simulink model "BlueROV2_Exp_Simu"  (R2023b)
settings: Solver=FixedStepAuto  StartTime=0.0  StopTime=120  FixedStep=dt  RelTol=1e-3
values from neighbouring files (symbols this model uses):
  Af = diag(ti)    [RM_param_AGF.m]
  B = [zeros(6,6) ... (first row only)    [EKF_param.m]
  Ballast_Force = Ballast_Compute(Ballast_Config)    [Integrate.m]    (also in init.m = Ballast_Term(Ballast_Config); init_NIF.m = [0; 0; 0; 0; 0; 0]; init_NIF2.m = [0; 0; Ballast_Term; 0]; init_ODE.m)
  dt = 0.1    [Integrate.m]    (also in init.m; init_NIF.m; init_NIF2.m; init_ODE.m)
  Gamma = diag(omega_is)    [RM_param_AGF.m]
  Gamma_o = dt*E    [EKF_param.m]
  H = [eye(6), zeros(6,6) zeros(6,6)]    [EKF_param.m]
  inv_M = inv(Param.MT)    [EKF_param.m]
  inv_Tb = inv(Tb)    [EKF_param.m]
  Kd = [155; 355; 8985; 1205; 1205; 1]    [Integrate.m]    (also in init.m = [1; 1; 1; 1; 1; 1]; init_NIF.m; init_NIF2.m; init_ODE.m)
  Ki = [45; 45; 10; 96; 96; 1]    [Integrate.m]    (also in init.m = [1; 1; 1; 1; 1; 1]; init_NIF.m; init_NIF2.m; init_ODE.m)
  Kp = [255; 545; 7095; 2420; 2375; 1]    [Integrate.m]    (also in init.m = [1; 1; 1; 1; 1; 1]; init_NIF.m; init_NIF2.m; init_ODE.m)
  lower_limit = -upper_limit    (= -30)    [Integrate.m]    (also in init.m; init_NIF.m; init_NIF2.m; init_ODE.m)
  Omega = diag(2*omega_is.*zeta_is)    [RM_param_AGF.m]
  Param = BlueROV2_param()    [Integrate.m]    (also in init.m; init_NIF.m; init_NIF2.m; init_ODE.m)
  Q = diag([0.1,0.1,pi/180,1e6,1e6,1e9])*10e3    [EKF_param.m]
  R = diag([0.00001,0.00001,0.00001,      0.01*pi/180,0.01*pi/180,0.01*pi/180])*10e-4    [EKF_param.m]
  T_alloc = Thrust_Allocation()    [Integrate.m]    (also in init_NIF.m; init_NIF2.m; init_ODE.m; init_ballast_checking.m)
  T_alloc_ps = pinv(T_alloc' * T_alloc + lambda * eye(size(T_alloc, 2))) * T_alloc'    [Integrate.m]    (also in init_NIF.m; init_NIF2.m; init_ODE.m; init_ballast_checking.m)
  Tether_Force = zeros(6,1)    [Integrate.m]    (also in init.m; init_NIF.m; init_NIF2.m; init_ODE.m)
  thrust_rate = 5    [Integrate.m]    (also in init.m; init_NIF.m; init_NIF2.m; init_ODE.m)
  upper_limit = 30    [Integrate.m]    (also in init.m; init_NIF.m; init_NIF2.m; init_ODE.m)
undefined symbols (not defined in the file or in its folder): model_val, Phi_ref, Psi_ref, Theta_ref, time_stamps_phi, time_stamps_psi, time_stamps_theta, time_stamps_x, time_stamps_y, time_stamps_z, time_val, X_ref, Y_ref, Z_ref
libraries: slpidlib x6
(part 1 of 2)
settings Model: Creator=goks  LastModifiedBy=HP

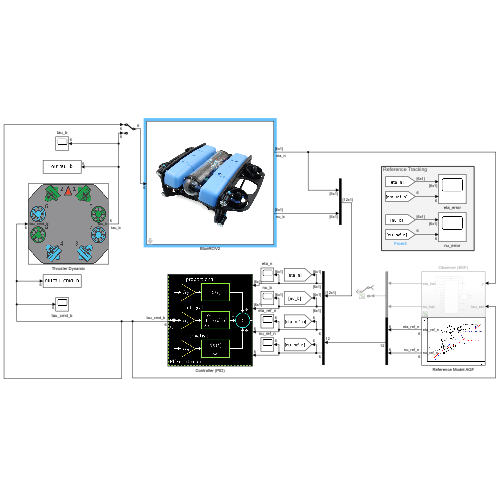
[thumbnail: Simulink's stored preview of the top-level diagram]
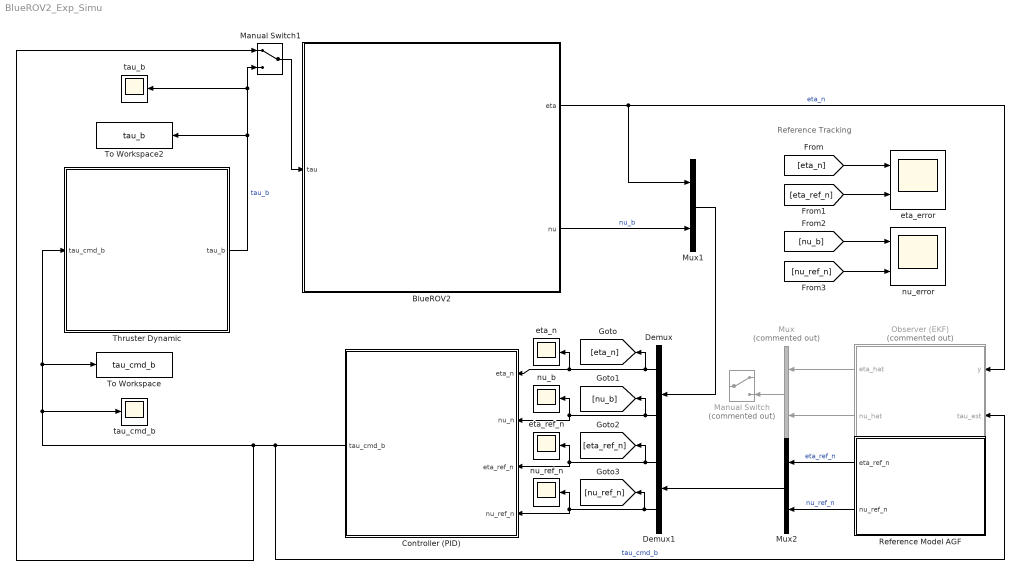
== system BlueROV2_Exp_Simu ==
  note: Reference Tracking
  BlueROV2 : Subsystem
      mask DialogControl DescTextVar Prompt: %<BlueROV2>
      mask Display: image('heavy-bluerov.jpg');
  Controller (PID) : Subsystem
      mask Display: image('pid.jpeg');
  Demux : Demux  Outputs=2
  Demux1 : Demux  Outputs=2
  Manual Switch : ManualSwitch  Commented=on
  Manual Switch1 : ManualSwitch
  Mux : Mux  Commented=on  Inputs=2
  Mux1 : Mux  Inputs=2
  Mux2 : Mux  Inputs=2
  Observer (EKF) : Subsystem  Commented=on
  Reference Model AGF : Subsystem
      mask Display: image('ref_traj_img.png');
  Thruster Dynamic : Subsystem
      mask Display: image('blueROV2_heavy_config.png');
  To Workspace : ToWorkspace  VariableName=tau_cmd_b  SampleTime=-1
  To Workspace2 : ToWorkspace  VariableName=tau_b  SampleTime=-1
  eta_error : Scope  NumInputPorts=2
  eta_n : Scope
  eta_ref_n : Scope
  nu_b : Scope
  nu_error : Scope  NumInputPorts=2
  nu_ref_n : Scope
  tau_b : Scope
  tau_cmd_b : Scope
  wires:
  BlueROV2/1(eta) -> Observer (EKF)/1(y), Mux1/1  "eta_n"
  Thruster Dynamic/1(tau_b) -> tau_b/1, Manual Switch1/2, To Workspace2/1  "tau_b"
  Controller (PID)/1(tau_cmd_b) -> Thruster Dynamic/1(tau_cmd_b), To Workspace/1, tau_cmd_b/1, Manual Switch1/1, Observer (EKF)/2(tau_est)  "tau_cmd_b"
  Observer (EKF)/1(eta_hat) -> Mux/1
  Observer (EKF)/2(nu_hat) -> Mux/2
  Mux/1 -> Manual Switch/2
  BlueROV2/2(nu) -> Mux1/2  "nu_b"
  Mux1/1 -> Demux/1
  Demux/1 -> Controller (PID)/1(eta_n), eta_n/1, [eta_n]
  Demux/2 -> Controller (PID)/2(nu_n), nu_b/1, [nu_b]
  Mux2/1 -> Demux1/1
  Demux1/1 -> Controller (PID)/3(eta_ref_n), eta_ref_n/1, [eta_ref_n]
  Demux1/2 -> Controller (PID)/4(nu_ref_n), nu_ref_n/1, [nu_ref_n]
  Manual Switch1/1 -> BlueROV2/1(tau)
  Reference Model AGF/1(eta_ref_n) -> Mux2/1  "eta_ref_n"
  Reference Model AGF/2(nu_ref_n) -> Mux2/2  "nu_ref_n"
  [eta_n] -> eta_error/1
  [eta_ref_n] -> eta_error/2
  [nu_b] -> nu_error/1
  [nu_ref_n] -> nu_error/2

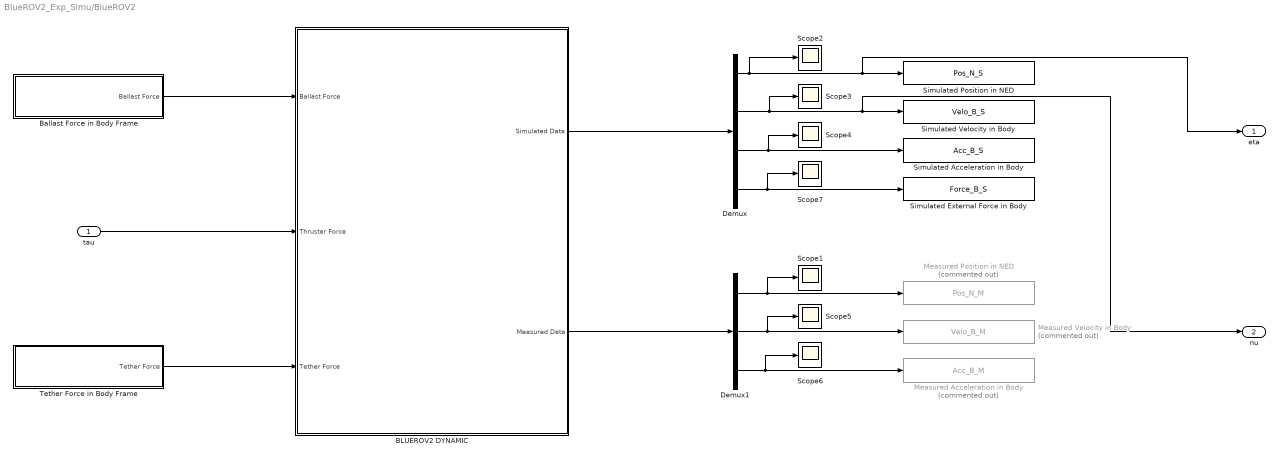
== system BlueROV2_Exp_Simu/BlueROV2 ==
  tau : Inport
  BLUEROV2 DYNAMIC : Subsystem
  Ballast Force in Body Frame : Subsystem
  Demux : Demux
  Demux1 : Demux  Outputs=3
  Measured Acceleration in Body : ToWorkspace  Commented=on  VariableName=Acc_B_M  SampleTime=-1
  Measured Position in NED : ToWorkspace  Commented=on  VariableName=Pos_N_M  SampleTime=-1
  Measured Velocity in Body : ToWorkspace  Commented=on  VariableName=Velo_B_M  SampleTime=-1
  Scope{1..7} (7 alike) : Scope
  Simulated Acceleration in Body : ToWorkspace  VariableName=Acc_B_S  SampleTime=-1
  Simulated External Force in Body : ToWorkspace  VariableName=Force_B_S  SampleTime=-1
  Simulated Position in NED : ToWorkspace  VariableName=Pos_N_S  SampleTime=-1
  Simulated Velocity in Body : ToWorkspace  VariableName=Velo_B_S  SampleTime=-1
  Tether Force in Body Frame : Subsystem
  eta : Outport
  nu : Outport  Port=2
  wires:
  Tether Force in Body Frame/1(Tether Force) -> BLUEROV2 DYNAMIC/3(Tether Force)
  Demux/2 -> nu/1, Simulated Velocity in Body/1, Scope3/1
  BLUEROV2 DYNAMIC/1(Simulated Data) -> Demux/1
  Demux1/1 -> Measured Position in NED/1, Scope1/1
  BLUEROV2 DYNAMIC/2(Measured Data) -> Demux1/1
  Ballast Force in Body Frame/1(Ballast Force) -> BLUEROV2 DYNAMIC/1(Ballast Force)
  Demux/1 -> eta/1, Simulated Position in NED/1, Scope2/1
  Demux/3 -> Simulated Acceleration in Body/1, Scope4/1
  tau/1 -> BLUEROV2 DYNAMIC/2(Thruster Force)
  Demux1/2 -> Measured Velocity in Body/1, Scope5/1
  Demux1/3 -> Scope6/1, Measured Acceleration in Body/1
  Demux/4 -> Scope7/1, Simulated External Force in Body/1

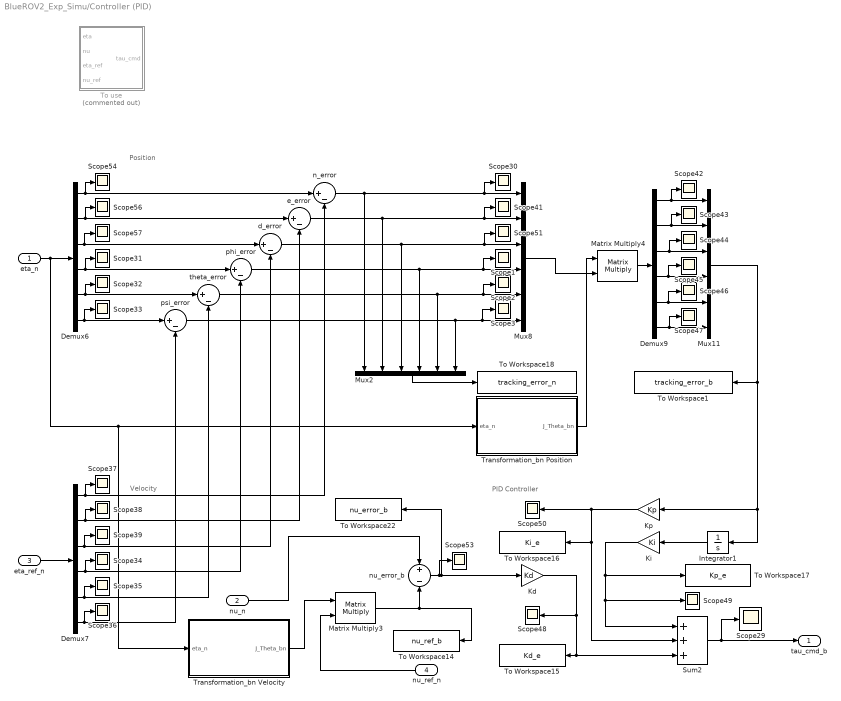
== system BlueROV2_Exp_Simu/Controller (PID) ==
  note: Velocity
  note: Position
  note: PID Controller
  eta_n : Inport
  nu_n : Inport  Port=2
  eta_ref_n : Inport  Port=3
  nu_ref_n : Inport  Port=4
  Demux6 : Demux  Outputs=6
  Demux7 : Demux  Outputs=6
  Demux9 : Demux  Outputs=6
  Integrator1 : Integrator
  Kd : Gain  Gain=Kd
  Ki : Gain  Gain=Ki
  Kp : Gain  Gain=Kp
  Matrix Multiply3 : Product  Multiplication=Matrix(*)
  Matrix Multiply4 : Product  Multiplication=Matrix(*)
  Mux11 : Mux  Inputs=6
  Mux2 : Mux  Inputs=6
  Mux8 : Mux  Inputs=6
  Scope{1..3,29..39,41..51,53..54,56..57} (29 alike) : Scope
  Sum2 : Sum  Inputs=+++
  To Workspace1 : ToWorkspace  VariableName=tracking_error_b  SampleTime=-1
  To Workspace14 : ToWorkspace  VariableName=nu_ref_b  SampleTime=-1
  To Workspace15 : ToWorkspace  VariableName=Kd_e  SampleTime=-1
  To Workspace16 : ToWorkspace  VariableName=Ki_e  SampleTime=-1
  To Workspace17 : ToWorkspace  VariableName=Kp_e  SampleTime=-1
  To Workspace18 : ToWorkspace  VariableName=tracking_error_n  SampleTime=-1
  To Workspace22 : ToWorkspace  VariableName=nu_error_b  SampleTime=-1
  To use : Subsystem  Commented=on
  Transformation_bn Position : MATLAB Function  TreatAsAtomicUnit=on
  Transformation_bn Velocity : MATLAB Function  TreatAsAtomicUnit=on
  d_error : Sum  Inputs=|+-
  e_error : Sum  Inputs=|+-
  n_error : Sum  Inputs=|+-
  nu_error_b : Sum  Inputs=+|-
  phi_error : Sum  Inputs=|+-
  psi_error : Sum  Inputs=|+-
  theta_error : Sum  Inputs=|+-
  tau_cmd_b : Outport
  wires:
  nu_ref_n/1 -> Matrix Multiply3/2
  Demux6/5 -> theta_error/1, Scope32/1
  Sum2/1 -> Scope29/1, tau_cmd_b/1
  Matrix Multiply4/1 -> Demux9/1
  Transformation_bn Velocity/1(J_Theta_bn) -> Matrix Multiply3/1
  n_error/1 -> Scope30/1, Mux8/1, Mux2/1
  Matrix Multiply3/1 -> nu_error_b/2, To Workspace14/1
  Mux2/1 -> To Workspace18/1
  Demux9/2 -> Scope43/1, Mux11/2
  Demux6/6 -> psi_error/1, Scope33/1
  Demux7/1 -> Scope37/1, n_error/2
  Integrator1/1 -> Ki/1
  eta_ref_n/1 -> Demux7/1
  Demux9/6 -> Scope47/1, Mux11/6
  Mux11/1 -> Integrator1/1, Kp/1, To Workspace1/1
  e_error/1 -> Scope41/1, Mux8/2, Mux2/2
  Demux9/3 -> Scope44/1, Mux11/3
  Mux8/1 -> Matrix Multiply4/2
  Demux7/4 -> Scope34/1, phi_error/2
  Demux6/4 -> phi_error/1, Scope31/1
  Demux6/2 -> Scope56/1, e_error/1
  d_error/1 -> Scope51/1, Mux8/3, Mux2/3
  Ki/1 -> Scope49/1, Sum2/1, To Workspace17/1
  Demux9/5 -> Scope46/1, Mux11/5
  Demux6/1 -> Scope54/1, n_error/1
  Kp/1 -> Scope50/1, To Workspace16/1, Sum2/2
  Demux9/4 -> Scope45/1, Mux11/4
  Kd/1 -> Sum2/3, To Workspace15/1, Scope48/1
  nu_error_b/1 -> Kd/1, To Workspace22/1, Scope53/1
  Transformation_bn Position/1(J_Theta_bn) -> Matrix Multiply4/1
  Demux7/6 -> Scope36/1, psi_error/2
  Demux9/1 -> Scope42/1, Mux11/1
  nu_n/1 -> nu_error_b/1
  Demux6/3 -> Scope57/1, d_error/1
  Demux7/2 -> Scope38/1, e_error/2
  phi_error/1 -> Scope1/1, Mux8/4, Mux2/4
  theta_error/1 -> Mux8/5, Scope2/1, Mux2/5
  psi_error/1 -> Scope3/1, Mux8/6, Mux2/6
  Demux7/3 -> d_error/2, Scope39/1
  Demux7/5 -> Scope35/1, theta_error/2
  eta_n/1 -> Transformation_bn Position/1(eta_n), Transformation_bn Velocity/1(eta_n), Demux6/1

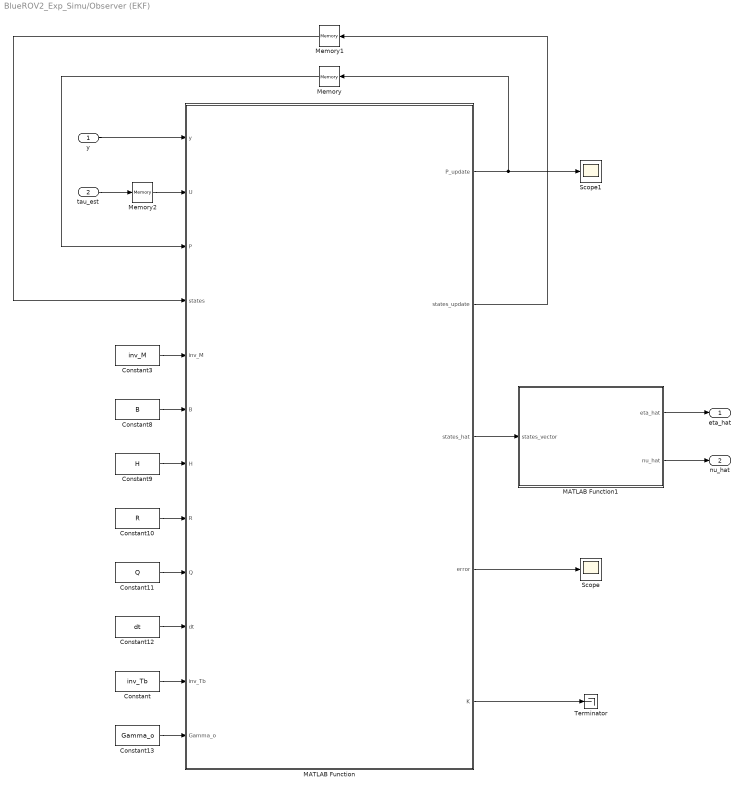
== system BlueROV2_Exp_Simu/Observer (EKF) ==
  y : Inport
  tau_est : Inport  Port=2
  Constant : Constant  Value=inv_Tb
  Constant10 : Constant  Value=R
  Constant11 : Constant  Value=Q
  Constant12 : Constant  Value=dt
  Constant13 : Constant  Value=Gamma_o
  Constant3 : Constant  Value=inv_M
  Constant8 : Constant  Value=B
  Constant9 : Constant  Value=H
  MATLAB Function : MATLAB Function  TreatAsAtomicUnit=on
  MATLAB Function1 : MATLAB Function  TreatAsAtomicUnit=on
  Memory : Memory  InitialCondition=eye(18)
  Memory1 : Memory  InitialCondition=zeros(18,1)
  Memory2 : Memory  InitialCondition=zeros(6,1)
  Scope : Scope
  Scope1 : Scope
  Terminator : Terminator
  eta_hat : Outport
  nu_hat : Outport  Port=2
  wires:
  y/1 -> MATLAB Function/1(y)
  Constant3/1 -> MATLAB Function/5(inv_M)
  Constant8/1 -> MATLAB Function/6(B)
  Constant9/1 -> MATLAB Function/7(H)
  Constant10/1 -> MATLAB Function/8(R)
  Constant11/1 -> MATLAB Function/9(Q)
  Constant12/1 -> MATLAB Function/10(dt)
  Constant/1 -> MATLAB Function/11(inv_Tb)
  Constant13/1 -> MATLAB Function/12(Gamma_o)
  MATLAB Function/1(P_update) -> Scope1/1, Memory/1
  Memory/1 -> MATLAB Function/3(P)
  MATLAB Function/2(states_update) -> Memory1/1
  Memory1/1 -> MATLAB Function/4(states)
  MATLAB Function/5(K) -> Terminator/1
  MATLAB Function/4(error) -> Scope/1
  MATLAB Function/3(states_hat) -> MATLAB Function1/1(states_vector)
  MATLAB Function1/1(eta_hat) -> eta_hat/1
  MATLAB Function1/2(nu_hat) -> nu_hat/1
  tau_est/1 -> Memory2/1
  Memory2/1 -> MATLAB Function/2(U)

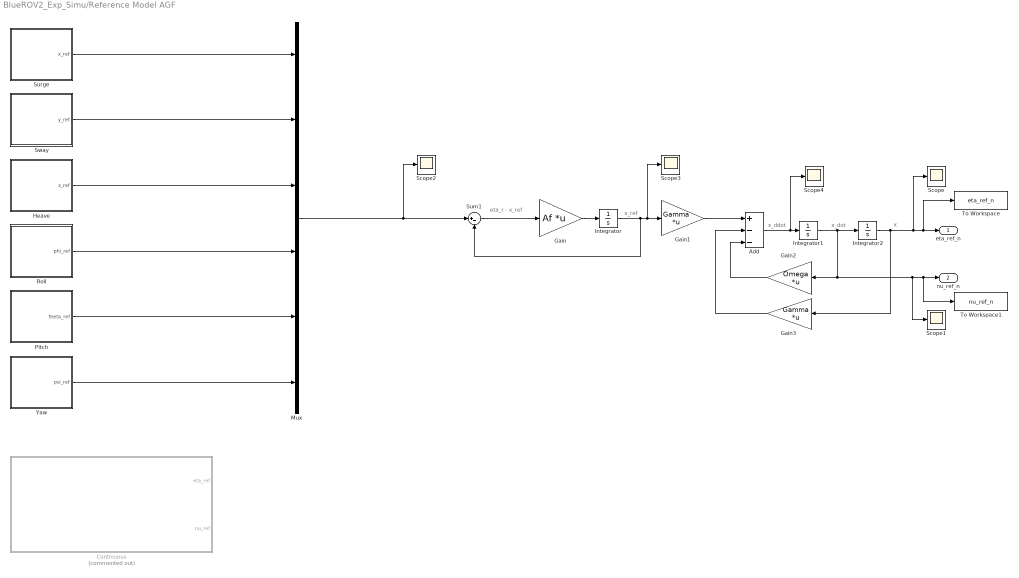
== system BlueROV2_Exp_Simu/Reference Model AGF ==
  note: x_dot
  note: eta_r - x_ref
  note: x
  note: x_ref
  note: x_ddot
  Add : Sum  Inputs=+--
  Continuous : Subsystem  Commented=on
  Gain : Gain  Gain=Af  Multiplication=Matrix(K*u)
  Gain1 : Gain  Gain=Gamma  Multiplication=Matrix(K*u)
  Gain2 : Gain  Gain=Omega  Multiplication=Matrix(K*u)
  Gain3 : Gain  Gain=Gamma  Multiplication=Matrix(K*u)
  Heave : Subsystem
  Integrator : Integrator
  Integrator1 : Integrator
  Integrator2 : Integrator
  Mux : Mux  Inputs=6
  Pitch : Subsystem
  Roll : Subsystem
  Scope{,1..4} (5 alike) : Scope
  Sum1 : Sum  Inputs=|+-
  Surge : Subsystem
  Sway : Subsystem
  To Workspace : ToWorkspace  VariableName=eta_ref_n  SampleTime=-1
  To Workspace1 : ToWorkspace  VariableName=nu_ref_n  SampleTime=-1
  Yaw : Subsystem
  eta_ref_n : Outport
  nu_ref_n : Outport  Port=2
  wires:
  Surge/1(x_ref) -> Mux/1
  Heave/1(z_ref) -> Mux/3
  Pitch/1(theta_ref) -> Mux/5
  Yaw/1(psi_ref) -> Mux/6
  Sway/1(y_ref) -> Mux/2
  Roll/1(phi_ref) -> Mux/4
  Gain1/1 -> Add/1
  Gain/1 -> Integrator/1
  Sum1/1 -> Gain/1
  Integrator1/1 -> Integrator2/1, To Workspace1/1, nu_ref_n/1, Scope1/1, Gain2/1
  Gain3/1 -> Add/2
  Integrator2/1 -> To Workspace/1, eta_ref_n/1, Scope/1, Gain3/1
  Gain2/1 -> Add/3
  Mux/1 -> Scope2/1, Sum1/1
  Integrator/1 -> Scope3/1, Gain1/1, Sum1/2
  Add/1 -> Scope4/1, Integrator1/1

== system BlueROV2_Exp_Simu/Thruster Dynamic ==
  tau_cmd_b : Inport
  Gain : Gain  Gain=T_alloc_ps  Multiplication=Matrix(K*u) (u vector)
  Gain1 : Gain  Gain=T_alloc  Multiplication=Matrix(K*u) (u vector)
  Manual Switch : ManualSwitch
  Saturation and Dynamics : Subsystem
      mask Display: image('t200-img.jpg');
  tau_b : Outport
  wires:
  Manual Switch/1 -> Gain1/1
  tau_cmd_b/1 -> Gain/1
  Saturation and Dynamics/1(Actual Thrust) -> Manual Switch/1
  Gain/1 -> Saturation and Dynamics/1(Commanded Thrust), Manual Switch/2
  Gain1/1 -> tau_b/1

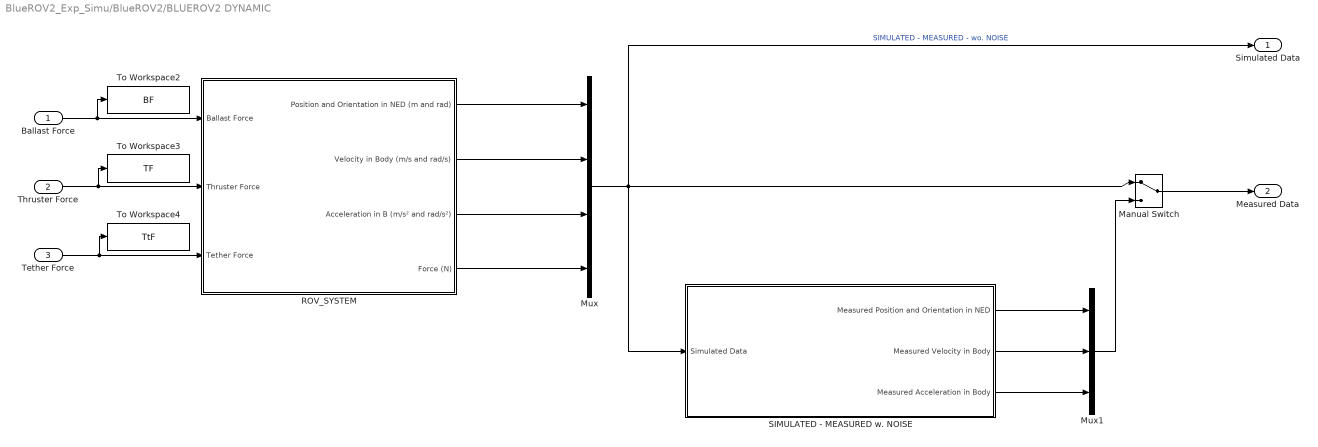
== system BlueROV2_Exp_Simu/BlueROV2/BLUEROV2 DYNAMIC ==
  Ballast Force : Inport
  Thruster Force : Inport  Port=2
  Tether Force : Inport  Port=3
  Manual Switch : ManualSwitch
  Mux : Mux
  Mux1 : Mux  Inputs=3
  ROV_SYSTEM : Subsystem
  SIMULATED - MEASURED w. NOISE : Subsystem
  To Workspace2 : ToWorkspace  VariableName=BF  SampleTime=-1
  To Workspace3 : ToWorkspace  VariableName=TF  SampleTime=-1
  To Workspace4 : ToWorkspace  VariableName=TtF  SampleTime=-1
  Simulated Data : Outport
  Measured Data : Outport  Port=2
  wires:
  ROV_SYSTEM/1(Position and Orientation in NED (m and rad)) -> Mux/1
  ROV_SYSTEM/2(Velocity in Body (m/s and rad/s)) -> Mux/2
  ROV_SYSTEM/3(Acceleration in B (m/s² and rad/s²)) -> Mux/3
  ROV_SYSTEM/4(Force (N)) -> Mux/4
  SIMULATED - MEASURED w. NOISE/2(Measured Velocity in Body) -> Mux1/2
  SIMULATED - MEASURED w. NOISE/1(Measured Position and Orientation in NED) -> Mux1/1
  SIMULATED - MEASURED w. NOISE/3(Measured Acceleration in Body) -> Mux1/3
  Mux/1 -> SIMULATED - MEASURED w. NOISE/1(Simulated Data), Manual Switch/1, Simulated Data/1  "SIMULATED - MEASURED - wo. NOISE"
  Manual Switch/1 -> Measured Data/1
  Mux1/1 -> Manual Switch/2
  Ballast Force/1 -> ROV_SYSTEM/1(Ballast Force), To Workspace2/1
  Thruster Force/1 -> ROV_SYSTEM/2(Thruster Force), To Workspace3/1
  Tether Force/1 -> To Workspace4/1, ROV_SYSTEM/3(Tether Force)

== system BlueROV2_Exp_Simu/BlueROV2/Ballast Force in Body Frame ==
  Ballast : Step  Time=0  Before=zeros(6,1)  After=Ballast_Force  SampleTime=0
  Scope : Scope
  Ballast Force : Outport
  wires:
  Ballast/1 -> Scope/1, Ballast Force/1

== system BlueROV2_Exp_Simu/BlueROV2/Tether Force in Body Frame ==
  Scope : Scope
  Tether : Step  Before=zeros(6,1)  After=Tether_Force  SampleTime=0
  Tether Force : Outport
  wires:
  Tether/1 -> Scope/1, Tether Force/1

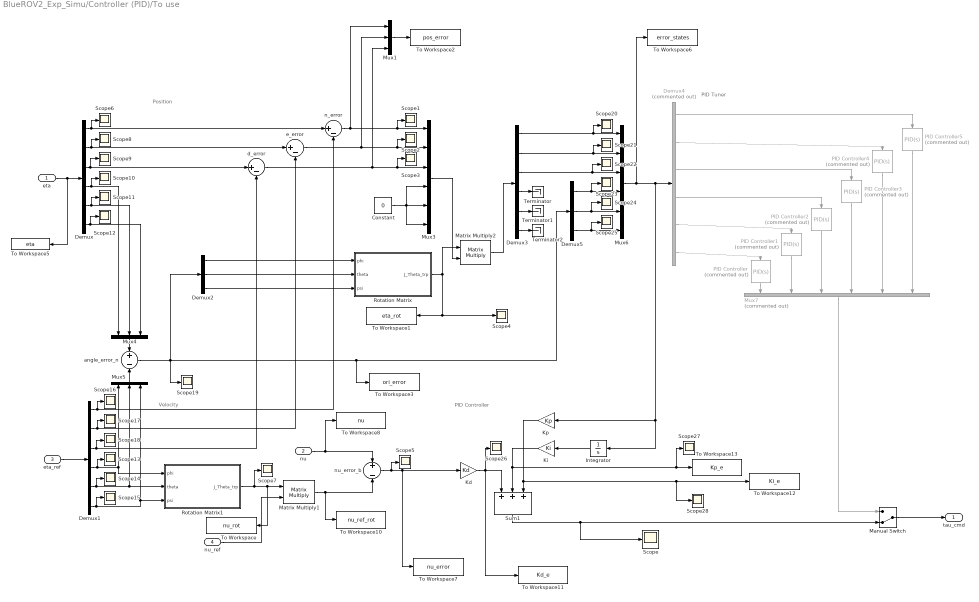
== system BlueROV2_Exp_Simu/Controller (PID)/To use ==
  note: PID Controller
  note: Velocity
  note: Position
  note: PID Tuner
  eta : Inport
  nu : Inport  Port=2
  eta_ref : Inport  Port=3
  nu_ref : Inport  Port=4
  Constant : Constant  Value=0
  Demux : Demux  Outputs=6
  Demux1 : Demux  Outputs=6
  Demux2 : Demux  Outputs=3
  Demux3 : Demux  Outputs=6
  Demux4 : Demux  Commented=on  Outputs=6
  Demux5 : Demux  Outputs=3
  Integrator : Integrator
  Kd : Gain  Gain=Kd
  Ki : Gain  Gain=Ki
  Kp : Gain  Gain=Kp
  Manual Switch : ManualSwitch  CurrentSetting=0
  Matrix Multiply1 : Product  Multiplication=Matrix(*)
  Matrix Multiply2 : Product  Multiplication=Matrix(*)
  Mux1 : Mux  Inputs=3
  Mux3 : Mux  Inputs=6
  Mux4 : Mux  Inputs=3
  Mux5 : Mux  Inputs=3
  Mux6 : Mux  Inputs=6
  Mux7 : Mux  Commented=on  Inputs=6
  PID Controller{,1,3..5} (5 alike) : slpidlib/PID Controller  Commented=on  Controller=PID  Form=Parallel  TimeDomain=Continuous-time  UseExternalTs=off  SampleTime=-1  IntegratorMethod=Forward Euler  FilterMethod=Forward Euler  ControllerParametersSource=internal  P=1  I=1  UseKiTs=off  D=0  N=100  UseFilter=on  TunerSelectOption=Transfer Function Based (PID Tuner App)  InitialConditionSource=internal  InitialConditionForIntegrator=0  InitialConditionForFilter=0  DifferentiatorICPrevScaledInput=0  ExternalReset=none  TrackingMode=off  Kt=1  LimitOutput=off  SatLimitsSource=internal  UpperSaturationLimit=inf  LowerSaturationLimit=-inf  LinearizeAsGain=on  AntiWindupMode=none  Kb=1  LimitIntegrator=off  UpperIntegratorSaturationLimit=inf  LowerIntegratorSaturationLimit=-inf  POutMin=[]  POutMax=[]  IOutMin=[]  IOutMax=[]  DOutMin=[]  DOutMax=[]  NOutMin=[]  NOutMax=[]  SumOutMin=[]  SumOutMax=[]  SaturationOutMin=[]  SaturationOutMax=[]  PParamMin=[]  PParamMax=[]  IParamMin=[]  IParamMax=[]  DParamMin=[]  DParamMax=[]  NParamMin=[]  NParamMax=[]  KbParamMin=[]  KbParamMax=[]  KtParamMin=[]  KtParamMax=[]  KbOutMin=[]  KbOutMax=[]  KtOutMin=[]  KtOutMax=[]  IntegratorOutMin=[]  IntegratorOutMax=[]  FilterOutMin=[]  FilterOutMax=[]  SumI1OutMin=[]  SumI1OutMax=[]  SumI2OutMin=[]  SumI2OutMax=[]  SumI3OutMin=[]  SumI3OutMax=[]  SumI4OutMin=[]  SumI4OutMax=[]  SumDOutMin=[]  SumDOutMax=[]  DifferentiatorOutMin=[]  DifferentiatorOutMax=[]  FilterDiffOutCoefMin=[]  FilterDiffOutCoefMax=[]  ReciprocalOutMin=[]  ReciprocalOutMax=[]  SumDenOutMin=[]  SumDenOutMax=[]  SumNumOutMin=[]  SumNumOutMax=[]  DivideOutMin=[]  DivideOutMax=[]  UdiffTsProdOutMin=[]  UdiffTsProdOutMax=[]  NTsProdOutMin=[]  NTsProdOutMax=[]  UintegralTsProdOutMin=[]  UintegralTsProdOutMax=[]  UngainTsProdOutMin=[]  UngainTsProdOutMax=[]  ClampingZeroOutDataTypeStr=Inherit: Inherit via back propagation  ClampingZeroOutMin=[]  ClampingZeroOutMax=[]  FilterDenConstantOutDataTypeStr=Inherit: Inherit via back propagation  FilterDenConstantOutMin=[]  FilterDenConstantOutMax=[]  PCopyOutDataTypeStr=Inherit: Inherit via back propagation  PCopyOutMin=[]  PCopyOutMax=[]  NCopyOutDataTypeStr=Inherit: Inherit via back propagation  NCopyOutMin=[]  NCopyOutMax=[]  IntegratorContinuousStateAttributes=''  IntegratorStateMustResolveToSignalObject=off  IntegratorRTWStateStorageClass=Auto  FilterContinuousStateAttributes=''  FilterStateMustResolveToSignalObject=off  FilterRTWStateStorageClass=Auto  ParallelPVariant=InternalParameters  IdealPVariant=Disabled  IVariant=InternalParameters  DVariant=InternalParameters  IntegratorVariant=Continuous  SatVariant=Disabled  AWVariant=Passthrough  PCopyVariant=Disabled  TRVariant=Disabled  FdbkBlocksVariant=Forward  IdealPFdbkVariant=Disabled  SatFdbkVariant=Disabled  DerivativeFilterVariant=ContFilter  NVariant=InternalParameters  NCopyVariant=Disabled  FilterICVariant=InternalICsFilter  IntegratorICVariant=InternalICs  ExternalResetVariant=Disabled  TRSumVariant=Passthrough  SumFdbkVariant=Disabled  SumVariant=Sum_PID  TsampFilterVariant=InternalTs  TsampNgainVariant=Passthrough  TsampIntegralVariant=Disabled_SignalSpec  ExternalSaturationOutDataTypeStr=Inherit: Same as second input
  PID Controller2 : slpidlib/PID Controller  Commented=on  Controller=PID  Form=Parallel  TimeDomain=Continuous-time  UseExternalTs=off  SampleTime=-1  IntegratorMethod=Forward Euler  FilterMethod=Forward Euler  ControllerParametersSource=internal  P=4.0249736275488e+41  I=3.47567522846608e+55  UseKiTs=off  D=4.27282188224195e+26  N=1.25606136924569e+18  UseFilter=on  TunerSelectOption=Transfer Function Based (PID Tuner App)  InitialConditionSource=internal  InitialConditionForIntegrator=0  InitialConditionForFilter=0  DifferentiatorICPrevScaledInput=0  ExternalReset=none  TrackingMode=off  Kt=1  LimitOutput=off  SatLimitsSource=internal  UpperSaturationLimit=inf  LowerSaturationLimit=-inf  LinearizeAsGain=on  AntiWindupMode=none  Kb=1  LimitIntegrator=off  UpperIntegratorSaturationLimit=inf  LowerIntegratorSaturationLimit=-inf  POutMin=[]  POutMax=[]  IOutMin=[]  IOutMax=[]  DOutMin=[]  DOutMax=[]  NOutMin=[]  NOutMax=[]  SumOutMin=[]  SumOutMax=[]  SaturationOutMin=[]  SaturationOutMax=[]  PParamMin=[]  PParamMax=[]  IParamMin=[]  IParamMax=[]  DParamMin=[]  DParamMax=[]  NParamMin=[]  NParamMax=[]  KbParamMin=[]  KbParamMax=[]  KtParamMin=[]  KtParamMax=[]  KbOutMin=[]  KbOutMax=[]  KtOutMin=[]  KtOutMax=[]  IntegratorOutMin=[]  IntegratorOutMax=[]  FilterOutMin=[]  FilterOutMax=[]  SumI1OutMin=[]  SumI1OutMax=[]  SumI2OutMin=[]  SumI2OutMax=[]  SumI3OutMin=[]  SumI3OutMax=[]  SumI4OutMin=[]  SumI4OutMax=[]  SumDOutMin=[]  SumDOutMax=[]  DifferentiatorOutMin=[]  DifferentiatorOutMax=[]  FilterDiffOutCoefMin=[]  FilterDiffOutCoefMax=[]  ReciprocalOutMin=[]  ReciprocalOutMax=[]  SumDenOutMin=[]  SumDenOutMax=[]  SumNumOutMin=[]  SumNumOutMax=[]  DivideOutMin=[]  DivideOutMax=[]  UdiffTsProdOutMin=[]  UdiffTsProdOutMax=[]  NTsProdOutMin=[]  NTsProdOutMax=[]  UintegralTsProdOutMin=[]  UintegralTsProdOutMax=[]  UngainTsProdOutMin=[]  UngainTsProdOutMax=[]  ClampingZeroOutDataTypeStr=Inherit: Inherit via back propagation  ClampingZeroOutMin=[]  ClampingZeroOutMax=[]  FilterDenConstantOutDataTypeStr=Inherit: Inherit via back propagation  FilterDenConstantOutMin=[]  FilterDenConstantOutMax=[]  PCopyOutDataTypeStr=Inherit: Inherit via back propagation  PCopyOutMin=[]  PCopyOutMax=[]  NCopyOutDataTypeStr=Inherit: Inherit via back propagation  NCopyOutMin=[]  NCopyOutMax=[]  IntegratorContinuousStateAttributes=''  IntegratorStateMustResolveToSignalObject=off  IntegratorRTWStateStorageClass=Auto  FilterContinuousStateAttributes=''  FilterStateMustResolveToSignalObject=off  FilterRTWStateStorageClass=Auto  ParallelPVariant=InternalParameters  IdealPVariant=Disabled  IVariant=InternalParameters  DVariant=InternalParameters  IntegratorVariant=Continuous  SatVariant=Disabled  AWVariant=Passthrough  PCopyVariant=Disabled  TRVariant=Disabled  FdbkBlocksVariant=Forward  IdealPFdbkVariant=Disabled  SatFdbkVariant=Disabled  DerivativeFilterVariant=ContFilter  NVariant=InternalParameters  NCopyVariant=Disabled  FilterICVariant=InternalICsFilter  IntegratorICVariant=InternalICs  ExternalResetVariant=Disabled  TRSumVariant=Passthrough  SumFdbkVariant=Disabled  SumVariant=Sum_PID  TsampFilterVariant=InternalTs  TsampNgainVariant=Passthrough  TsampIntegralVariant=Disabled_SignalSpec  ExternalSaturationOutDataTypeStr=Inherit: Same as second input
  Rotation Matrix : MATLAB Function  TreatAsAtomicUnit=on
  Rotation Matrix1 : MATLAB Function  TreatAsAtomicUnit=on
  Scope{,1..28} (29 alike) : Scope
  Sum1 : Sum  Inputs=+++
  Terminator : Terminator
  Terminator1 : Terminator
  Terminator2 : Terminator
  To Workspace : ToWorkspace  VariableName=nu_rot  SampleTime=-1
  To Workspace1 : ToWorkspace  VariableName=eta_rot  SampleTime=-1
  To Workspace10 : ToWorkspace  VariableName=nu_ref_rot  SampleTime=-1
  To Workspace11 : ToWorkspace  VariableName=Kd_e  SampleTime=-1
  To Workspace12 : ToWorkspace  VariableName=Ki_e  SampleTime=-1
  To Workspace13 : ToWorkspace  VariableName=Kp_e  SampleTime=-1
  To Workspace2 : ToWorkspace  VariableName=pos_error  SampleTime=-1
  To Workspace3 : ToWorkspace  VariableName=ori_error  SampleTime=-1
  To Workspace5 : ToWorkspace  VariableName=eta  SampleTime=-1
  To Workspace6 : ToWorkspace  VariableName=error_states  SampleTime=-1
  To Workspace7 : ToWorkspace  VariableName=nu_error  SampleTime=-1
  To Workspace8 : ToWorkspace  VariableName=nu  SampleTime=-1
  angle_error_n : Sum  Inputs=+|-
  d_error : Sum  Inputs=|+-
  e_error : Sum  Inputs=|+-
  n_error : Sum  Inputs=|+-
  nu_error_b : Sum  Inputs=+|-
  tau_cmd : Outport
  wires:
  Kp/1 -> Sum1/3, Scope28/1, To Workspace12/1
  Demux1/3 -> Scope18/1, d_error/2
  Demux4/2 -> PID Controller4/1
  Mux6/1 -> To Workspace6/1, Kp/1, Integrator/1, Demux4/1
  eta/1 -> To Workspace5/1, Demux/1
  Demux3/3 -> Scope22/1, Mux6/3
  nu_ref/1 -> Matrix Multiply1/2
  Matrix Multiply2/1 -> Demux3/1
  PID Controller3/1 -> Mux7/4
  Sum1/1 -> Manual Switch/2, Scope/1
  Matrix Multiply1/1 -> nu_error_b/2, To Workspace10/1
  Manual Switch/1 -> tau_cmd/1
  Demux/5 -> Scope11/1, Mux4/2
  nu/1 -> nu_error_b/1, To Workspace8/1
  PID Controller/1 -> Mux7/1
  Demux/3 -> Scope9/1, d_error/1
  Demux/2 -> Scope8/1, e_error/1
  Rotation Matrix1/1(J_Theta_trp) -> Scope7/1, To Workspace/1, Matrix Multiply1/1
  e_error/1 -> Mux1/2, Scope2/1, Mux3/2
  PID Controller1/1 -> Mux7/2
  Demux/6 -> Scope12/1, Mux4/3
  Demux3/1 -> Scope20/1, Mux6/1
  Ki/1 -> Sum1/2, Scope27/1, To Workspace13/1
  PID Controller2/1 -> Mux7/3
  Demux4/6 -> PID Controller/1
  Mux4/1 -> angle_error_n/1
  Demux4/4 -> PID Controller2/1
  Kd/1 -> Scope26/1, To Workspace11/1, Sum1/1
  Demux4/3 -> PID Controller3/1
  Demux4/1 -> PID Controller5/1
  Mux7/1 -> Manual Switch/1
  PID Controller4/1 -> Mux7/5
  Demux5/1 -> Scope23/1, Mux6/4
  Demux1/5 -> Scope14/1, Rotation Matrix1/2(theta), Mux5/2
  nu_error_b/1 -> Scope5/1, To Workspace7/1, Kd/1
  Demux3/6 -> Terminator2/1
  n_error/1 -> Scope1/1, Mux3/1, Mux1/1
  Demux1/6 -> Scope15/1, Mux5/3, Rotation Matrix1/3(psi)
  Demux3/5 -> Terminator1/1
  Demux3/4 -> Terminator/1
  Integrator/1 -> Ki/1
  Demux2/2 -> Rotation Matrix/2(theta)
  Demux1/1 -> Scope16/1, n_error/2
  eta_ref/1 -> Demux1/1
  Mux1/1 -> To Workspace2/1
  Demux1/4 -> Scope13/1, Rotation Matrix1/1(phi), Mux5/1
  Demux3/2 -> Scope21/1, Mux6/2
  Demux5/2 -> Scope24/1, Mux6/5
  Demux/4 -> Scope10/1, Mux4/1
  Demux5/3 -> Scope25/1, Mux6/6
  d_error/1 -> Mux1/3, Scope3/1, Mux3/3
  Mux3/1 -> Matrix Multiply2/2
  Demux2/1 -> Rotation Matrix/1(phi)
  Mux5/1 -> angle_error_n/2
  Demux1/2 -> Scope17/1, e_error/2
  Demux2/3 -> Rotation Matrix/3(psi)
  PID Controller5/1 -> Mux7/6
  Constant/1 -> Mux3/6, Mux3/4, Mux3/5
  angle_error_n/1 -> Demux2/1, Scope19/1, Demux5/1, To Workspace3/1
  Rotation Matrix/1(J_Theta_trp) -> Scope4/1, To Workspace1/1, Matrix Multiply2/1
  Demux4/5 -> PID Controller1/1
  Demux/1 -> Scope6/1, n_error/1

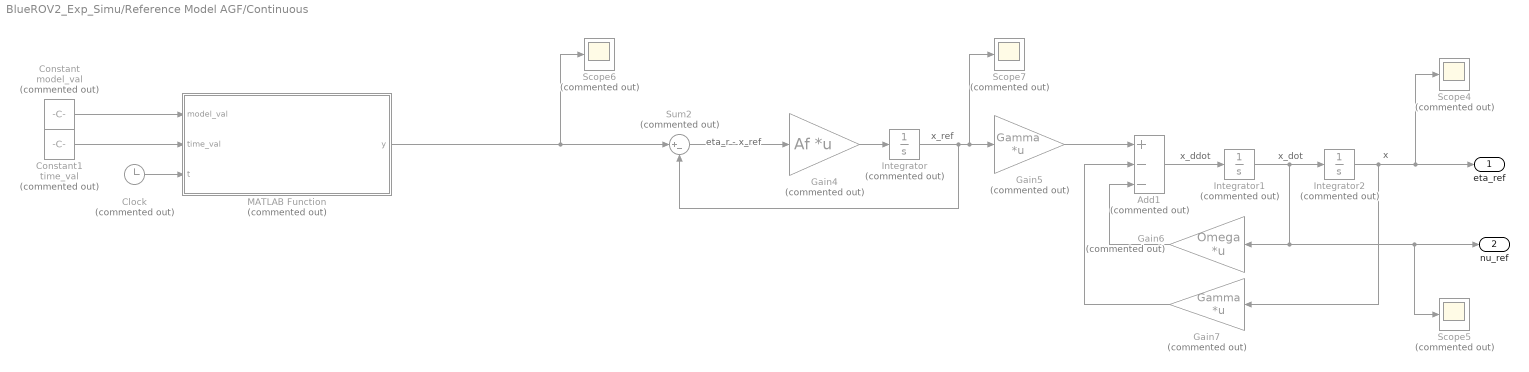
== system BlueROV2_Exp_Simu/Reference Model AGF/Continuous ==
  note: x_dot
  note: x_ddot
  note: x
  note: eta_r - x_ref
  note: x_ref
  Add1 : Sum  Commented=on  Inputs=+--
  Clock : Clock  Commented=on
  Constant : Constant  Commented=on  Value=model_val
  Constant1 : Constant  Commented=on  Value=time_val
  Gain4 : Gain  Commented=on  Gain=Af  Multiplication=Matrix(K*u)
  Gain5 : Gain  Commented=on  Gain=Gamma  Multiplication=Matrix(K*u)
  Gain6 : Gain  Commented=on  Gain=Omega  Multiplication=Matrix(K*u)
  Gain7 : Gain  Commented=on  Gain=Gamma  Multiplication=Matrix(K*u)
  Integrator : Integrator  Commented=on
  Integrator1 : Integrator  Commented=on
  Integrator2 : Integrator  Commented=on
  MATLAB Function : MATLAB Function  Commented=on  TreatAsAtomicUnit=on
  Scope{4..7} (4 alike) : Scope  Commented=on
  Sum2 : Sum  Commented=on  Inputs=|+-
  eta_ref : Outport
  nu_ref : Outport  Port=2
  wires:
  Gain7/1 -> Add1/2
  Clock/1 -> MATLAB Function/3(t)
  Gain6/1 -> Add1/3
  Integrator/1 -> Scope7/1, Gain5/1, Sum2/2
  Add1/1 -> Integrator1/1
  Constant/1 -> MATLAB Function/1(model_val)
  Gain4/1 -> Integrator/1
  Gain5/1 -> Add1/1
  Integrator1/1 -> Integrator2/1, nu_ref/1, Scope5/1, Gain6/1
  MATLAB Function/1(y) -> Scope6/1, Sum2/1
  Sum2/1 -> Gain4/1
  Integrator2/1 -> eta_ref/1, Scope4/1, Gain7/1
  Constant1/1 -> MATLAB Function/2(time_val)

== system BlueROV2_Exp_Simu/Reference Model AGF/Heave ==
  Clock1 : Clock
  Constant2 : Constant  Value=Z_ref
  Constant3 : Constant  Value=time_stamps_z
  MATLAB Function1 : MATLAB Function  TreatAsAtomicUnit=on
  z_ref : Outport
  wires:
  Constant3/1 -> MATLAB Function1/2(time_stamps)
  MATLAB Function1/1(ref) -> z_ref/1
  Clock1/1 -> MATLAB Function1/3(t)
  Constant2/1 -> MATLAB Function1/1(val_checkpoints)

== system BlueROV2_Exp_Simu/Reference Model AGF/Pitch ==
  Clock1 : Clock
  Constant2 : Constant  Value=Theta_ref
  Constant3 : Constant  Value=time_stamps_theta
  MATLAB Function1 : MATLAB Function  TreatAsAtomicUnit=on
  theta_ref : Outport
  wires:
  Constant3/1 -> MATLAB Function1/2(time_stamps)
  MATLAB Function1/1(ref) -> theta_ref/1
  Clock1/1 -> MATLAB Function1/3(t)
  Constant2/1 -> MATLAB Function1/1(val_checkpoints)

== system BlueROV2_Exp_Simu/Reference Model AGF/Roll ==
  Clock1 : Clock
  Constant2 : Constant  Value=Phi_ref
  Constant3 : Constant  Value=time_stamps_phi
  MATLAB Function1 : MATLAB Function  TreatAsAtomicUnit=on
  phi_ref : Outport
  wires:
  Constant3/1 -> MATLAB Function1/2(time_stamps)
  MATLAB Function1/1(ref) -> phi_ref/1
  Clock1/1 -> MATLAB Function1/3(t)
  Constant2/1 -> MATLAB Function1/1(val_checkpoints)

== system BlueROV2_Exp_Simu/Reference Model AGF/Surge ==
  Clock1 : Clock
  Constant2 : Constant  Value=X_ref
  Constant3 : Constant  Value=time_stamps_x
  MATLAB Function1 : MATLAB Function  TreatAsAtomicUnit=on
  x_ref : Outport
  wires:
  MATLAB Function1/1(ref) -> x_ref/1
  Clock1/1 -> MATLAB Function1/3(t)
  Constant2/1 -> MATLAB Function1/1(val_checkpoints)
  Constant3/1 -> MATLAB Function1/2(time_stamps)

== system BlueROV2_Exp_Simu/Reference Model AGF/Sway ==
  Clock1 : Clock
  Constant2 : Constant  Value=Y_ref
  Constant3 : Constant  Value=time_stamps_y
  MATLAB Function1 : MATLAB Function  TreatAsAtomicUnit=on
  y_ref : Outport
  wires:
  Constant3/1 -> MATLAB Function1/2(time_stamps)
  MATLAB Function1/1(ref) -> y_ref/1
  Clock1/1 -> MATLAB Function1/3(t)
  Constant2/1 -> MATLAB Function1/1(val_checkpoints)

== system BlueROV2_Exp_Simu/Reference Model AGF/Yaw ==
  Clock1 : Clock
  Constant2 : Constant  Value=Psi_ref
  Constant3 : Constant  Value=time_stamps_psi
  MATLAB Function1 : MATLAB Function  TreatAsAtomicUnit=on
  psi_ref : Outport
  wires:
  Constant3/1 -> MATLAB Function1/2(time_stamps)
  MATLAB Function1/1(ref) -> psi_ref/1
  Clock1/1 -> MATLAB Function1/3(t)
  Constant2/1 -> MATLAB Function1/1(val_checkpoints)

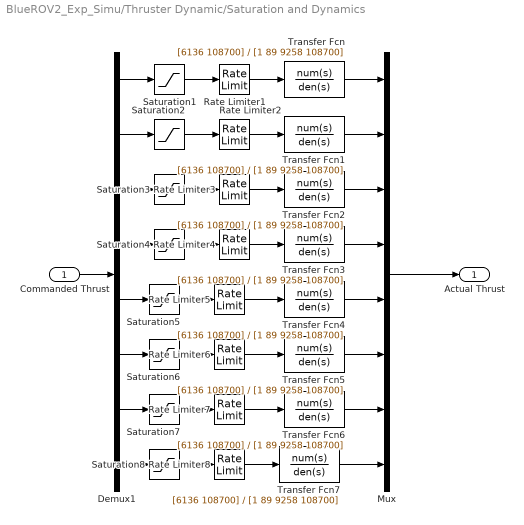
== system BlueROV2_Exp_Simu/Thruster Dynamic/Saturation and Dynamics ==
  Commanded Thrust : Inport
  Demux1 : Demux  Outputs=8
  Mux : Mux  Inputs=8
  Rate Limiter{1..8} (8 alike) : RateLimiter  RisingSlewLimit=thrust_rate  FallingSlewLimit=-thrust_rate  SampleTimeMode=inherited
  Saturation{1..8} (8 alike) : Saturate  UpperLimit=upper_limit  LowerLimit=lower_limit
  Transfer Fcn{,1..7} (8 alike) : TransferFcn  Numerator=[6136 108700]  Denominator=[1 89 9258 108700]
  Actual Thrust : Outport
  wires:
  Demux1/4 -> Saturation4/1
  Rate Limiter7/1 -> Transfer Fcn6/1
  Saturation2/1 -> Rate Limiter2/1
  Demux1/5 -> Saturation5/1
  Demux1/2 -> Saturation2/1
  Demux1/8 -> Saturation8/1
  Demux1/3 -> Saturation3/1
  Rate Limiter1/1 -> Transfer Fcn/1
  Saturation1/1 -> Rate Limiter1/1
  Demux1/6 -> Saturation6/1
  Demux1/7 -> Saturation7/1
  Rate Limiter3/1 -> Transfer Fcn2/1
  Rate Limiter2/1 -> Transfer Fcn1/1
  Saturation8/1 -> Rate Limiter8/1
  Rate Limiter5/1 -> Transfer Fcn4/1
  Rate Limiter6/1 -> Transfer Fcn5/1
  Saturation5/1 -> Rate Limiter5/1
  Saturation3/1 -> Rate Limiter3/1
  Saturation6/1 -> Rate Limiter6/1
  Saturation7/1 -> Rate Limiter7/1
  Demux1/1 -> Saturation1/1
  Rate Limiter4/1 -> Transfer Fcn3/1
  Saturation4/1 -> Rate Limiter4/1
  Rate Limiter8/1 -> Transfer Fcn7/1
  Commanded Thrust/1 -> Demux1/1
  Mux/1 -> Actual Thrust/1
  Transfer Fcn/1 -> Mux/1
  Transfer Fcn1/1 -> Mux/2
  Transfer Fcn2/1 -> Mux/3
  Transfer Fcn3/1 -> Mux/4
  Transfer Fcn4/1 -> Mux/5
  Transfer Fcn5/1 -> Mux/6
  Transfer Fcn6/1 -> Mux/7
  Transfer Fcn7/1 -> Mux/8

== system BlueROV2_Exp_Simu/BlueROV2/BLUEROV2 DYNAMIC/ROV_SYSTEM ==
  Ballast Force : Inport
  Thruster Force : Inport  Port=2
  Tether Force : Inport  Port=3
  DYNAMIC SOLVER : Subsystem
  Position and Orientation in NED (m and rad) : Outport
  Velocity in Body (m/s and rad/s) : Outport  Port=2
  Acceleration in B (m/s² and rad/s²) : Outport  Port=3
  Force (N) : Outport  Port=4
  wires:
  DYNAMIC SOLVER/2(Velocity in Body (m/s and rad/s)) -> Velocity in Body (m/s and rad/s)/1
  DYNAMIC SOLVER/1(Position and Orientation in NED (m and rad)) -> Position and Orientation in NED (m and rad)/1
  DYNAMIC SOLVER/3(Acceleration in B (m/s² and rad/s²)) -> Acceleration in B (m/s² and rad/s²)/1
  Thruster Force/1 -> DYNAMIC SOLVER/2(Thruster Force), Force (N)/1
  Ballast Force/1 -> DYNAMIC SOLVER/1(Ballast Force)
  Tether Force/1 -> DYNAMIC SOLVER/3(Tether Force)

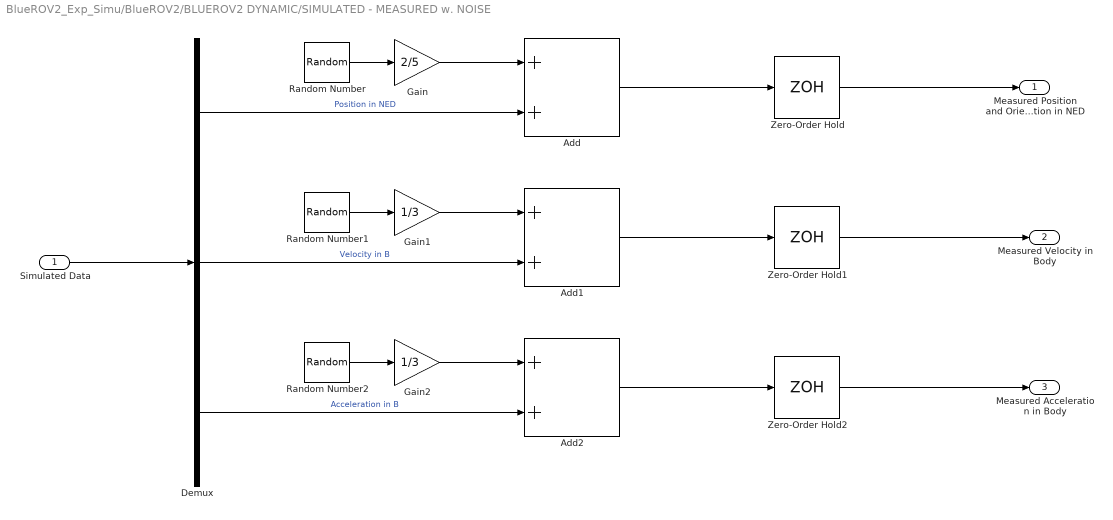
== system BlueROV2_Exp_Simu/BlueROV2/BLUEROV2 DYNAMIC/SIMULATED - MEASURED w. NOISE ==
  Simulated Data : Inport
  Add : Sum
  Add1 : Sum
  Add2 : Sum
  Demux : Demux  Outputs=3
  Gain : Gain  Gain=2/5
  Gain1 : Gain  Gain=1/3
  Gain2 : Gain  Gain=1/3
  Random Number : RandomNumber  Variance=0.01  SampleTime=dt
  Random Number1 : RandomNumber  Variance=0.01  SampleTime=dt
  Random Number2 : RandomNumber  Variance=0.01  SampleTime=dt
  Zero-Order Hold : ZeroOrderHold  SampleTime=-1
  Zero-Order Hold1 : ZeroOrderHold  SampleTime=-1
  Zero-Order Hold2 : ZeroOrderHold  SampleTime=-1
  Measured Position and Orientation in NED : Outport
  Measured Velocity in Body : Outport  Port=2
  Measured Acceleration in Body : Outport  Port=3
  wires:
  Simulated Data/1 -> Demux/1
  Demux/1 -> Add/2  "Position in NED"
  Random Number/1 -> Gain/1
  Gain/1 -> Add/1
  Random Number1/1 -> Gain1/1
  Demux/2 -> Add1/2  "Velocity in B"
  Gain1/1 -> Add1/1
  Random Number2/1 -> Gain2/1
  Demux/3 -> Add2/2  "Acceleration in B"
  Gain2/1 -> Add2/1
  Add/1 -> Zero-Order Hold/1
  Add1/1 -> Zero-Order Hold1/1
  Add2/1 -> Zero-Order Hold2/1
  Zero-Order Hold/1 -> Measured Position and Orientation in NED/1
  Zero-Order Hold1/1 -> Measured Velocity in Body/1
  Zero-Order Hold2/1 -> Measured Acceleration in Body/1

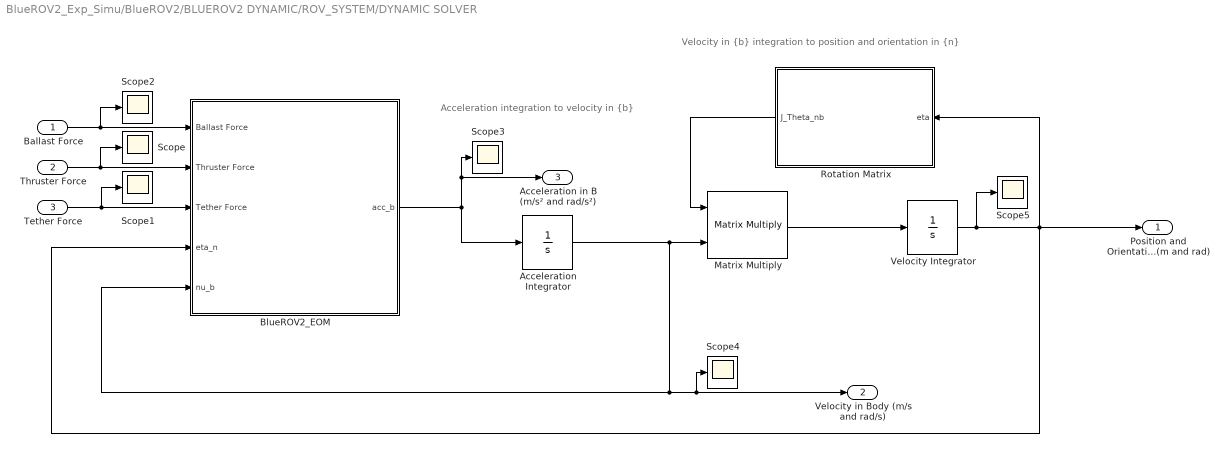
== system BlueROV2_Exp_Simu/BlueROV2/BLUEROV2 DYNAMIC/ROV_SYSTEM/DYNAMIC SOLVER ==
  note: Velocity in {b} integration to position and orientation in {n}
  note: Acceleration integration to velocity in {b}
  Ballast Force : Inport
  Thruster Force : Inport  Port=2
  Tether Force : Inport  Port=3
  Acceleration Integrator : Integrator  InitialCondition=Param.IC.Velo
  BlueROV2_EOM : Subsystem
  Matrix Multiply : Product  Multiplication=Matrix(*)
  Rotation Matrix : MATLAB Function  TreatAsAtomicUnit=on
  Scope{,1..5} (6 alike) : Scope
  Velocity Integrator : Integrator  InitialCondition=Param.IC.Pos
  Position and Orientation in NED (m and rad) : Outport
  Velocity in Body (m/s and rad/s) : Outport  Port=2
  Acceleration in B (m/s² and rad/s²) : Outport  Port=3
  wires:
  Thruster Force/1 -> BlueROV2_EOM/2(Thruster Force), Scope/1
  Rotation Matrix/1(J_Theta_nb) -> Matrix Multiply/1
  Matrix Multiply/1 -> Velocity Integrator/1
  Ballast Force/1 -> Scope2/1, BlueROV2_EOM/1(Ballast Force)
  BlueROV2_EOM/1(acc_b) -> Acceleration Integrator/1, Scope3/1, Acceleration in B (m/s² and rad/s²)/1
  Tether Force/1 -> BlueROV2_EOM/3(Tether Force), Scope1/1
  Velocity Integrator/1 -> BlueROV2_EOM/4(eta_n), Position and Orientation in NED (m and rad)/1, Rotation Matrix/1(eta), Scope5/1
  Acceleration Integrator/1 -> BlueROV2_EOM/5(nu_b), Scope4/1, Velocity in Body (m/s and rad/s)/1, Matrix Multiply/2

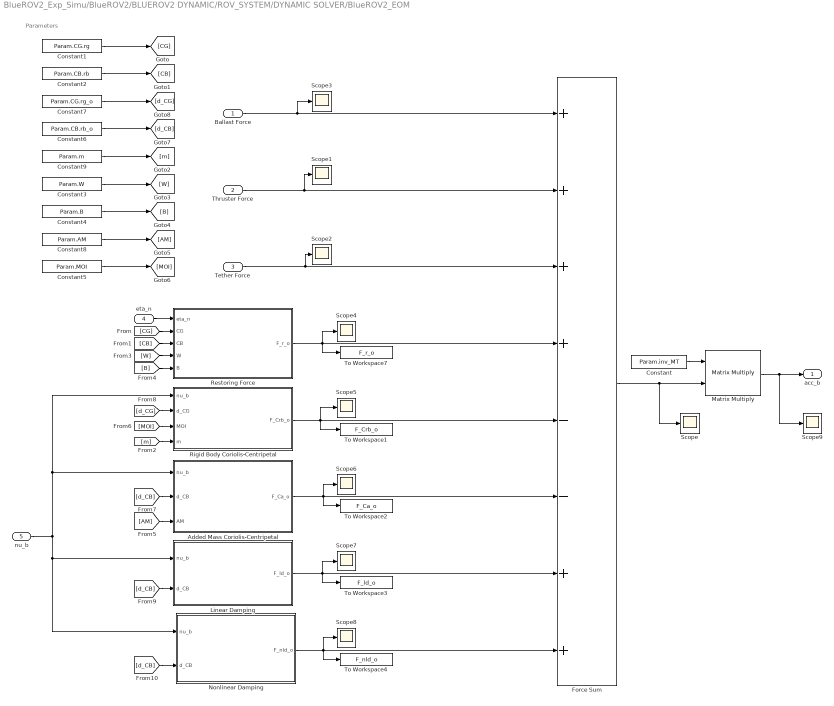
== system BlueROV2_Exp_Simu/BlueROV2/BLUEROV2 DYNAMIC/ROV_SYSTEM/DYNAMIC SOLVER/BlueROV2_EOM ==
  note: Parameters
  Ballast Force : Inport
  Thruster Force : Inport  Port=2
  Tether Force : Inport  Port=3
  eta_n : Inport  Port=4
  nu_b : Inport  Port=5
  Added Mass Coriolis-Centripetal : MATLAB Function  TreatAsAtomicUnit=on
  Constant : Constant  Value=Param.inv_MT
  Constant1 : Constant  Value=Param.CG.rg
  Constant2 : Constant  Value=Param.CB.rb
  Constant3 : Constant  Value=Param.W
  Constant4 : Constant  Value=Param.B
  Constant5 : Constant  Value=Param.MOI
  Constant6 : Constant  Value=Param.CB.rb_o
  Constant7 : Constant  Value=Param.CG.rg_o
  Constant8 : Constant  Value=Param.AM
  Constant9 : Constant  Value=Param.m
  Force Sum : Sum  Inputs=++++--++
  Linear Damping : MATLAB Function  TreatAsAtomicUnit=on
  Matrix Multiply : Product  Multiplication=Matrix(*)
  Nonlinear Damping : MATLAB Function  TreatAsAtomicUnit=on
  Restoring Force : MATLAB Function  TreatAsAtomicUnit=on
  Rigid Body Coriolis-Centripetal : MATLAB Function  TreatAsAtomicUnit=on
  Scope{,1..9} (10 alike) : Scope
  To Workspace1 : ToWorkspace  VariableName=F_Crb_o  SampleTime=-1
  To Workspace2 : ToWorkspace  VariableName=F_Ca_o  SampleTime=-1
  To Workspace3 : ToWorkspace  VariableName=F_ld_o  SampleTime=-1
  To Workspace4 : ToWorkspace  VariableName=F_nld_o  SampleTime=-1
  To Workspace7 : ToWorkspace  VariableName=F_r_o  SampleTime=-1
  acc_b : Outport
  wires:
  eta_n/1 -> Restoring Force/1(eta_n)
  nu_b/1 -> Nonlinear Damping/1(nu_b), Linear Damping/1(nu_b), Rigid Body Coriolis-Centripetal/1(nu_b), Added Mass Coriolis-Centripetal/1(nu_b)
  Force Sum/1 -> Scope/1, Matrix Multiply/2
  Constant/1 -> Matrix Multiply/1
  Matrix Multiply/1 -> Scope9/1, acc_b/1
  Ballast Force/1 -> Scope3/1, Force Sum/1
  Thruster Force/1 -> Scope1/1, Force Sum/2
  Tether Force/1 -> Scope2/1, Force Sum/3
  Restoring Force/1(F_r_o) -> To Workspace7/1, Force Sum/4, Scope4/1
  Rigid Body Coriolis-Centripetal/1(F_Crb_o) -> Scope5/1, To Workspace1/1, Force Sum/5
  Added Mass Coriolis-Centripetal/1(F_Ca_o) -> To Workspace2/1, Scope6/1, Force Sum/6
  Linear Damping/1(F_ld_o) -> To Workspace3/1, Scope7/1, Force Sum/7
  Nonlinear Damping/1(F_nld_o) -> Scope8/1, To Workspace4/1, Force Sum/8
  Constant1/1 -> [CG]
  Constant2/1 -> [CB]
  Constant6/1 -> [d_CB]
  Constant7/1 -> [d_CG]
  Constant9/1 -> [m]
  Constant3/1 -> [W]
  Constant4/1 -> [B]
  Constant8/1 -> [AM]
  Constant5/1 -> [MOI]
  [CG] -> Restoring Force/2(CG)
  [CB] -> Restoring Force/3(CB)
  [W] -> Restoring Force/4(W)
  [B] -> Restoring Force/5(B)
  [d_CG] -> Rigid Body Coriolis-Centripetal/2(d_CG)
  [m] -> Rigid Body Coriolis-Centripetal/4(m)
  [MOI] -> Rigid Body Coriolis-Centripetal/3(MOI)
  [d_CB] -> Added Mass Coriolis-Centripetal/2(d_CB)
  [AM] -> Added Mass Coriolis-Centripetal/3(AM)
  [d_CB] -> Linear Damping/2(d_CB)
  [d_CB] -> Nonlinear Damping/2(d_CB)

== matlab function BlueROV2_Exp_Simu/Controller (PID)/Transformation_bn Velocity ==
  data: eta_n input; J_Theta_bn output
function J_Theta_bn  = Transform_bn(eta_n)
%%%%%%%%%%%%%%%%%%%%%%%%%%%%%%%%%%%%%%%%%%%%%%%%%%%%%%%%%%%%%%%%%%%%%%%%%%%
% Command                                                                 %
%                                                                         %
% Compute the Jacobian from {b} to {n}                                    %
%                                                                         %
% For 6-DOF Equations:                                                    %
% [ndot = Jacobian(n_theta) * v]                                          %
% -ndot = velocity expressed in NED frame                                 %
% -n_theta = rotational part of position vector                           %
% - v = velocity expressed in Body frame                                  %
%                                                                         %
% Argument:                                                               %
% eta     : Input positional vector                                       %
%                                                                         %
% Created:      27.09.2023	Andreas Sitorus                               %
%                                                                         %
%%%%%%%%%%%%%%%%%%%%%%%%%%%%%%%%%%%%%%%%%%%%%%%%%%%%%%%%%%%%%%%%%%%%%%%%%%%
%% Get the angular velocity
phi = eta_n(4);       % Rolling angle
theta = eta_n(5);     % Pitching angle
psi = eta_n(6);       % Yaw angle

%% Linear Velocity Transformation Matrix
% Element
r11 = cos(psi) * cos(theta);
r12 = -sin(psi) * cos(phi) + cos(psi) * sin(theta) * sin(phi);
r13 = sin(psi) * sin(phi) + cos(psi) * cos(phi) * sin(theta);
r21 = sin(psi) * cos(theta);
r22 = cos(psi) * cos(phi) + sin(phi) * sin(theta) * sin(psi);
r23 = -cos(psi) * sin(phi) + sin(theta) * sin(psi) * cos(phi);
r31 = -sin(theta);
r32 = cos(theta) * sin(phi);
r33 = cos(theta) * cos(phi);

% Rotation Matrix (from {b} to {n})
R_Theta_nb = [r11 r12 r13;
              r21 r22 r23;
              r31 r32 r33];

%% Angular Velocity Transformation Matrix
% Element
t11 = 1;
t12 = sin(phi) * tan(theta);
t13 = cos(phi) * tan(theta);
t21 = 0;
t22 = cos(phi);
t23 = -sin(phi);
t31 = 0;
t32 = sin(phi) / cos(theta);
t33 = cos(phi) / cos(theta);

% Angular Velocity Rotation Matrix (from {b} to {n})
T_Theta_nb = [t11 t12 t13;
              t21 t22 t23;
              t31 t32 t33];

%% Jacobian
J_Theta_nb = [R_Theta_nb  zeros(3);
              zeros(3) T_Theta_nb];
J_Theta_bn = J_Theta_nb';
end

== matlab function BlueROV2_Exp_Simu/Reference Model AGF/Heave/MATLAB Function1 ==
  data: val_checkpoints input; time_stamps input; ref output; t input
function ref = generate_step_signal(val_checkpoints, time_stamps, t)
    % Initialize output signal
    ref = zeros(size(t));

    % Iterate through set points
    for i = 1:length(val_checkpoints)
        value = val_checkpoints(i);
        time = time_stamps(i);

        % Generate step signal
        ref(t >= time) = value;
    end
end

== matlab function BlueROV2_Exp_Simu/Reference Model AGF/Pitch/MATLAB Function1 ==
  data: val_checkpoints input; time_stamps input; ref output; t input
function ref = generate_step_signal(val_checkpoints, time_stamps, t)
    % Initialize output signal
    ref = zeros(size(t));

    % Iterate through set points
    for i = 1:length(val_checkpoints)
        value = val_checkpoints(i);
        time = time_stamps(i);

        % Generate step signal
        ref(t >= time) = value;
    end
end

== matlab function BlueROV2_Exp_Simu/Reference Model AGF/Roll/MATLAB Function1 ==
  data: val_checkpoints input; time_stamps input; ref output; t input
function ref = generate_step_signal(val_checkpoints, time_stamps, t)
    % Initialize output signal
    ref = zeros(size(t));

    % Iterate through set points
    for i = 1:length(val_checkpoints)
        value = val_checkpoints(i);
        time = time_stamps(i);

        % Generate step signal
        ref(t >= time) = value;
    end
end

== matlab function BlueROV2_Exp_Simu/Reference Model AGF/Sway/MATLAB Function1 ==
  data: val_checkpoints input; time_stamps input; ref output; t input
function ref = generate_step_signal(val_checkpoints, time_stamps, t)
    % Initialize output signal
    ref = zeros(size(t));

    % Iterate through set points
    for i = 1:length(val_checkpoints)
        value = val_checkpoints(i);
        time = time_stamps(i);

        % Generate step signal
        ref(t >= time) = value;
    end
end

== matlab function BlueROV2_Exp_Simu/Reference Model AGF/Yaw/MATLAB Function1 ==
  data: val_checkpoints input; time_stamps input; ref output; t input
function ref = generate_step_signal(val_checkpoints, time_stamps, t)
    % Initialize output signal
    ref = zeros(size(t));

    % Iterate through set points
    for i = 1:length(val_checkpoints)
        value = val_checkpoints(i);
        time = time_stamps(i);

        % Generate step signal
        ref(t >= time) = value;
    end
end

== matlab function BlueROV2_Exp_Simu/BlueROV2/BLUEROV2 DYNAMIC/ROV_SYSTEM/DYNAMIC SOLVER/BlueROV2_EOM/Rigid Body Coriolis-Centripetal ==
  data: nu_b input; F_Crb_o output; d_CG input; MOI input; m input
function F_Crb_o    = Coriolis_Centripetal_RB_Force(nu_b, d_CG, MOI, m)
%% Coriolis-Centripetal Forces
% Velocity
u = nu_b(1);
v = nu_b(2);
w = nu_b(3);
p = nu_b(4);
q = nu_b(5);
r = nu_b(6);

% Distance from CG to CO
% Defined as d_CG

% Transformed Velocity
V_t_g = H_(-d_CG) * nu_b;  % 6DOF Velocity, expressed in CG

% MOI
Ixx = MOI(1);
Iyy = MOI(2);
Izz = MOI(3);

% CC-Rigid Body
% Described in Body frame, at Center of Gravity

Crb11 = zeros(3); 
Crb12 = [0 m*w -m*v;
         -m*w 0 m*u;
         m*v -m*u 0];
Crb21 = Crb12;
Crb22 = [0 -Izz*r -Iyy*q;
         Izz*r 0 Ixx*p;
         Iyy*q -Ixx*p 0];

Crb = [Crb11 Crb12;
       Crb21 Crb22]; % Rigid Body Coriolis Force Matrix, at Center of Gravity

% Force
F_Crb_o = (H_(d_CG))' * Crb * V_t_g;

% For debugging
% F_Crb_o = Crb * nu_b;
% F_Crb_o = zeros(6,1);
end

== matlab function BlueROV2_Exp_Simu/Reference Model AGF/Continuous/MATLAB Function ==
  data: model_val input; time_val input; y output; t input
function y = generate_step_signal(model_val, time_val, t)
    % Initialize output signal
    y = zeros(size(t));

    % Iterate through set points
    for i = 1:length(model_val)
        value = model_val(i);
        time = time_val(i);

        % Generate step signal
        y(t >= time) = value;
    end
end

== matlab function BlueROV2_Exp_Simu/Reference Model AGF/Surge/MATLAB Function1 ==
  data: val_checkpoints input; time_stamps input; ref output; t input
function ref = generate_step_signal(val_checkpoints, time_stamps, t)
    % Initialize output signal
    ref = zeros(size(t));

    % Iterate through set points
    for i = 1:length(val_checkpoints)
        value = val_checkpoints(i);
        time = time_stamps(i);

        % Generate step signal
        ref(t >= time) = value;
    end
end

== matlab function BlueROV2_Exp_Simu/BlueROV2/BLUEROV2 DYNAMIC/ROV_SYSTEM/DYNAMIC SOLVER/BlueROV2_EOM/Added Mass Coriolis-Centripetal ==
  data: nu_b input; F_Ca_o output; d_CB input; AM input
function F_Ca_o    = Coriolis_Centripetal_AM_Force(nu_b, d_CB, AM)
%% Coriolis-Centripetal Forces
% Velocity
u = nu_b(1);
v = nu_b(2);
w = nu_b(3);
p = nu_b(4);
q = nu_b(5);
r = nu_b(6);

% Distance from CB to CO
% Defined as d_CB

% Transformed Velocity
V_t_b = H_(-d_CB) * nu_b;  % 6DOF Velocity, expressed in CB

% Added Mass Coefficient
Xud = AM(1);
Yvd = AM(2);
Zwd = AM(3);
Kpd = AM(4);
Mqd = AM(5);
Nrd = AM(6);

% CC-Added Mass
% Described in Body frame, at Center of Buoyancy
Ca11 = zeros(3);
Ca12 = [0 -Zwd*w Yvd*v;
        Zwd*w 0 -Xud*u;
        -Yvd*v Xud*u 0];
Ca21 = Ca12;
Ca22 = [0 -Nrd*r Mqd*q;
        Nrd*r 0 -Kpd*p;
        -Mqd*q Kpd*p 0];

Ca = [Ca11 Ca12;
      Ca21 Ca22]; % Added mass Coriolis Force Matrix, at Center of Buoyancy

% Force
F_Ca_o = (H_(d_CB))' * Ca * V_t_b;

% For debugging
% F_Ca_o = Ca * nu_b;
% F_Ca_o = zeros(6,1);
end

== matlab function BlueROV2_Exp_Simu/BlueROV2/BLUEROV2 DYNAMIC/ROV_SYSTEM/DYNAMIC SOLVER/BlueROV2_EOM/Linear Damping ==
  data: F_ld_o output; nu_b input; d_CB input
function F_ld_o  = Linear_Damping(nu_b, d_CB)
% %% Linear Damping Forces
% % Distance from CB to CO
% % Defined as d_CB

% Transformed Velocity
V_t_b = H_(-d_CB) * nu_b;  % 6DOF Velocity, expressed in CB

% Linear Damping Coefficient
Xu_l = 13.7;    % N.s/m
Yv_l = 0;       % N.s/m
Zw_l = 33.0;    % N.s/m
Kp_l = 0;       % N.s/m
Mq_l = 0.8;     % N.s/m
Nr_l = 0;       % N.s/m

% Linear Damping Matrix
L_Damping_Matrix = [Xu_l Yv_l Zw_l Kp_l Mq_l Nr_l];

% Force
F_ld_o = (H_(d_CB)) * diag(L_Damping_Matrix) * V_t_b; 

% For debugging
% F_ld_o = -diag(L_Damping_Matrix) * nu_b; 
% F_ld_o = zeros(6,1); 
end

== matlab function BlueROV2_Exp_Simu/BlueROV2/BLUEROV2 DYNAMIC/ROV_SYSTEM/DYNAMIC SOLVER/BlueROV2_EOM/Nonlinear Damping ==
  data: F_nld_o output; nu_b input; d_CB input
function F_nld_o = Nonlinear_Damping_forces(nu_b, d_CB)
%% Nonlinear Damping Forces
% Velocity
u = nu_b(1);
v = nu_b(2);
w = nu_b(3);
p = nu_b(4);
q = nu_b(5);
r = nu_b(6);

% Distance from CB to CO
% Defined as d_CB

% Transformed Velocity
V_t_b = H_(-d_CB) * nu_b;  % 6DOF Velocity, expressed in CB

% Nonlinear Damping Coefficient
Xu_nl = 141.0;  % N.s2/m2
Yv_nl = 217.0;  % N.s2/m2
Zw_nl = 190.0;  % N.s2/m2
Kp_nl = 1.192;  % N.s2/m2
Mq_nl = 0.470;  % N.s2/m2
Nr_nl = 1.500;  % N.s2/m2

% Nonlinear Damping Matrix
NL_Damping_Coeff = diag([Xu_nl Yv_nl Zw_nl Kp_nl Mq_nl Nr_nl]) * abs(V_t_b);

% Force
F_nld_o = (H_(d_CB))' * diag(NL_Damping_Coeff) * V_t_b;

% For debugging
% F_nld_o = diag(NL_Damping_Coeff) * abs(nu_b);
% F_nld_o = zeros(6,1);
end

== matlab function BlueROV2_Exp_Simu/BlueROV2/BLUEROV2 DYNAMIC/ROV_SYSTEM/DYNAMIC SOLVER/BlueROV2_EOM/Restoring Force ==
  data: eta_n input; F_r_o output; CG input; CB input; W input; B input
function F_r_o   = Restoring_Force(eta_n, CG, CB, W, B)
%% Restoring Forces
% Described in Body Frame, at Center of Gravity. ALREADY FOR THE LEFT HAND SIDE
% % Orientation
% phi = eta_n(4);
% theta = eta_n(5);
% 
% % Gravity
% xg = CG(1);
% yg = CG(2);
% zg = CG(3);
% rb_g = [xg; yg; zg];
% 
% % Buoyancy
% xb = CB(1);
% yb = CB(2);
% zb = CB(3);
% rb_b = [xb; yb; zb];

% Force
Fg_n = [0; 0; W];
Fb_n = -[0; 0; B];

F_r_o = [Rot_bn(eta_n) * Fg_n + Rot_bn(eta_n) * Fb_n;
         cross(CG, Rot_bn(eta_n) * Fg_n) + cross(CB, Rot_bn(eta_n) * Fb_n)];

% % Force
% F_r_o = [(W - B)*sin(theta);
%       -(W - B)*cos(theta)*sin(phi);
%       -(W - B)*cos(theta)*cos(phi);
%       -(yg*W - yb*B)*cos(theta)*cos(phi) + (zg*W - zb*B)*cos(theta)*sin(phi);
%       (zg*W - zb*B)*sin(theta) + (xg*W - xb*B)*cos(theta)*cos(phi);
%       -(xg*W - xb*B)*cos(theta)*sin(phi) - (yg*W - yb*B)*sin(theta)];

% For debugging
% F_r_o = zeros(6,1);
end

== matlab function BlueROV2_Exp_Simu/BlueROV2/BLUEROV2 DYNAMIC/ROV_SYSTEM/DYNAMIC SOLVER/Rotation Matrix ==
  data: eta input; J_Theta_nb output
function J_Theta_nb = Transform_bn(eta)

J_Theta_nb = Jacobian(eta);

end
